simulink model "System_Stability_Evaluation"  (R2024a)
settings: Solver=VariableStepAuto  StartTime=0.0  StopTime=10.0  RelTol=1e-3
undefined symbols (not defined in the file or in its folder): sigbuilder_block
libraries: cstblocks x3
settings Model: Creator=marin  LastModifiedBy=marin

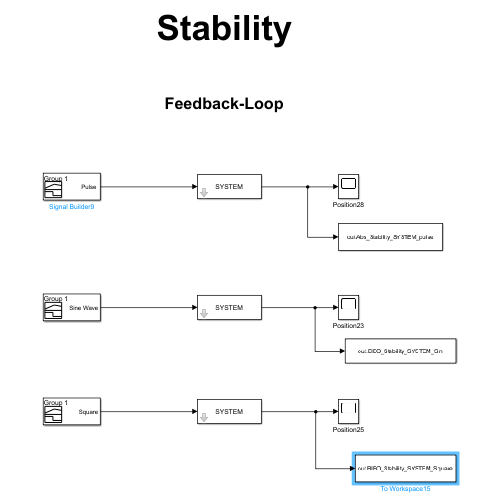
[thumbnail: Simulink's stored preview of the top-level diagram]
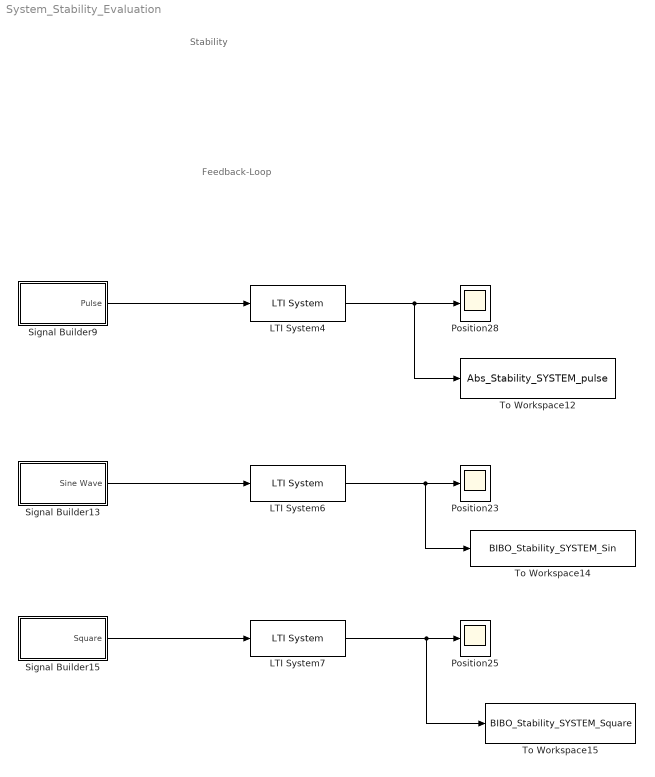
== system System_Stability_Evaluation ==
  note: Stability
  note: Feedback-Loop
  LTI System4 : cstblocks/LTI System  sys=SYSTEM  IC=[]  PadeOrder=0
  LTI System6 : cstblocks/LTI System  sys=SYSTEM  IC=[]  PadeOrder=0
  LTI System7 : cstblocks/LTI System  sys=SYSTEM  IC=[]  PadeOrder=0
  Position23 : Scope
  Position25 : Scope
  Position28 : Scope
  Signal Builder13 : Subsystem  Tag=STV Subsys  LoadFcn=sigbuilder_block('load');  StartFcn=sigbuilder_block('start');  StopFcn=sigbuilder_block('stop');  ClipboardFcn=sigbuilder_block('clipboard');  mask(Sigbuilder block){tuvar=[0:10]}
      mask help: Simulink:masks:SigbuilderBlock_MD
      mask init:
      | if ~strcmp(get_param(bdroot(gcbh),'SimulationStatus'),'stopped') tuvar = sigbuilder_block('maskInit'); end
      settings: CopyFcn=sigbuilder_block('copy');  DeleteFcn=sigbuilder_block('delete');  ModelCloseFcn=sigbuilder_block('modelClose');  PreSaveFcn=sigbuilder_block('preSave');  PauseFcn=sigbuilder_block('pause');  ContinueFcn=sigbuilder_block('continue');  NameChangeFcn=sigbuilder_block('namechange');  OpenFcn=sigbuilder_block('open',[404 117.5 550.5 362.5 ]);  CloseFcn=sigbuilder_block('close');
      mask Display: plot(0, 0, 100, 100,[2, 2, 32, 32, 2], [68, 8, 8, 68, 68],[32, 2], [38, 38], [32, 19, 2],[53, 60, 44], [32, 17, 17, 2],[16, 16, 31, 31]);txt = getActiveGroup(gcbh);text(2, 100, txt,'verticalAlignment', 'top');
  Signal Builder15 : Subsystem  Tag=STV Subsys  LoadFcn=sigbuilder_block('load');  StartFcn=sigbuilder_block('start');  StopFcn=sigbuilder_block('stop');  ClipboardFcn=sigbuilder_block('clipboard');  mask(Sigbuilder block){tuvar=[0:10]}
      mask help: Simulink:masks:SigbuilderBlock_MD
      mask init:
      | if ~strcmp(get_param(bdroot(gcbh),'SimulationStatus'),'stopped') tuvar = sigbuilder_block('maskInit'); end
      settings: CopyFcn=sigbuilder_block('copy');  DeleteFcn=sigbuilder_block('delete');  ModelCloseFcn=sigbuilder_block('modelClose');  PreSaveFcn=sigbuilder_block('preSave');  PauseFcn=sigbuilder_block('pause');  ContinueFcn=sigbuilder_block('continue');  NameChangeFcn=sigbuilder_block('namechange');  OpenFcn=sigbuilder_block('open',[404 117.5 550.5 362.5 ]);  CloseFcn=sigbuilder_block('close');
      mask Display: plot(0, 0, 100, 100,[2, 2, 32, 32, 2], [68, 8, 8, 68, 68],[32, 2], [38, 38], [32, 19, 2],[53, 60, 44], [32, 17, 17, 2],[16, 16, 31, 31]);txt = getActiveGroup(gcbh);text(2, 100, txt,'verticalAlignment', 'top');
  Signal Builder9 : Subsystem  Tag=STV Subsys  LoadFcn=sigbuilder_block('load');  StartFcn=sigbuilder_block('start');  StopFcn=sigbuilder_block('stop');  ClipboardFcn=sigbuilder_block('clipboard');  mask(Sigbuilder block){tuvar=[0:10]}
      mask help: Simulink:masks:SigbuilderBlock_MD
      mask init:
      | if ~strcmp(get_param(bdroot(gcbh),'SimulationStatus'),'stopped') tuvar = sigbuilder_block('maskInit'); end
      settings: CopyFcn=sigbuilder_block('copy');  DeleteFcn=sigbuilder_block('delete');  ModelCloseFcn=sigbuilder_block('modelClose');  PreSaveFcn=sigbuilder_block('preSave');  PauseFcn=sigbuilder_block('pause');  ContinueFcn=sigbuilder_block('continue');  NameChangeFcn=sigbuilder_block('namechange');  OpenFcn=sigbuilder_block('open',[404 117.5 550.5 362.5 ]);  CloseFcn=sigbuilder_block('close');
      mask Display: plot(0, 0, 100, 100,[2, 2, 32, 32, 2], [68, 8, 8, 68, 68],[32, 2], [38, 38], [32, 19, 2],[53, 60, 44], [32, 17, 17, 2],[16, 16, 31, 31]);txt = getActiveGroup(gcbh);text(2, 100, txt,'verticalAlignment', 'top');
  To Workspace12 : ToWorkspace  VariableName=Abs_Stability_SYSTEM_pulse  SampleTime=-1
  To Workspace14 : ToWorkspace  VariableName=BIBO_Stability_SYSTEM_Sin  SampleTime=-1
  To Workspace15 : ToWorkspace  VariableName=BIBO_Stability_SYSTEM_Square  SampleTime=-1
  wires:
  LTI System4/1 -> Position28/1, To Workspace12/1
  Signal Builder9/1("Pulse ") -> LTI System4/1
  Signal Builder15/1(Square) -> LTI System7/1
  LTI System7/1 -> Position25/1, To Workspace15/1
  LTI System6/1 -> Position23/1, To Workspace14/1
  Signal Builder13/1(Sine Wave) -> LTI System6/1

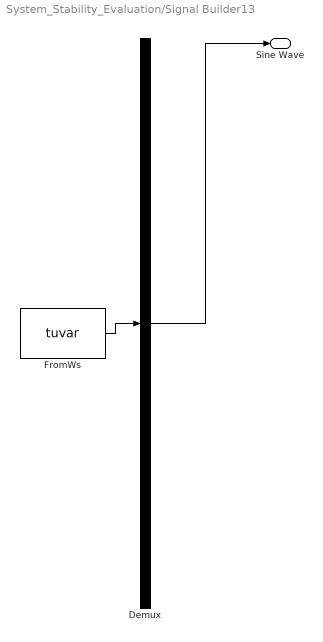
== system System_Stability_Evaluation/Signal Builder13 ==
  Demux : Demux  Tag=STV Demux  Outputs=1
      settings: DisplayOption=none
  FromWs : FromWorkspace  Tag=STV FromWs  VariableName=tuvar
      SigBuilderData=|
      | common.afterFinalStr = 'Extrapolate'
      | common.sampleTime = 0
      | dataSet.timeRange = [0 10]
      | dataSet.name = 'Group 1'
      | sbobj.Groups.Name = 'Group 1'
      | sbobj.Groups.Signals.Name = 'Sine Wave'
      | sbobj.Groups.Signals.XData = [0 0.111111111111 0.222222222222 0.333333333333 0.444444444444 0.555555555556 0.666666666667 0.777777777778 0.888888888889 1 1.11111111111 1.22222222222 1.33333333333 1.44444444444 1.55555555556 1.66666666667 1.77777777778 1.88888888889 2 2.11111111111 2.22222222222 2.33333333333 2.44444444444 2.55555555556 2.66666666667 2.77777777778 2.88888888889 3 3.11111111111 3.22222222222 3.33333333333 3.44444444444 3.55555555556 3.66666666667 3.77777777778 3.88888888889 4 4.11111111111 4.22222222222 4.33333333333 4.44444444444 4.55555555556 4.66666666667 4.77777777778 4.88888888889 5 5.11111111111 5.22222222222 5.33333333333 5.44444444444 5.55555555556 5.66666666667 5.77777777778 5.88888888889 6 6.11111111111 6.22222222222 6.33333333333 6.44444444444 6.55555555556 6.66666666667 6.77777777778 6.88888888889 7 7.11111111111 7.22222222222 7.33333333333 7.44444444444 7.55555555556 7.66666666667 7.77777777778 7.88888888889 8 8.11111111111 8.22222222222 8.33333333333 8.44444444444 8.55555555556 8.66666666667 8.77777777778 8.88888888889 9 9.11111111111 9.22222222222 9.33333333333 9.44444444444 9.55555555556 9.66666666667 9.77777777778 9.88888888889 10]
      | sbobj.Groups.Signals.YData = [1 1.64278760969 1.98480775301 1.86602540378 1.34202014333 0.657979856674 0.133974596216 0.0151922469878 0.357212390313 1 1.64278760969 1.98480775301 1.86602540378 1.34202014333 0.657979856674 0.133974596216 0.0151922469878 0.357212390313 1 1.64278760969 1.98480775301 1.86602540378 1.34202014333 0.657979856674 0.133974596216 0.0151922469878 0.357212390313 1 1.64278760969 1.98480775301 1.86602540378 1.34202014333 0.657979856674 0.133974596216 0.0151922469878 0.357212390313 1 1.64278760969 1.98480775301 1.86602540378 1.34202014333 0.657979856674 0.133974596216 0.0151922469878 0.357212390313 1 1.64278760969 1.98480775301 1.86602540378 1.34202014333 0.657979856674 0.133974596216 0.0151922469878 0.357212390313 1 1.64278760969 1.98480775301 1.86602540378 1.34202014333 0.657979856674 0.133974596216 0.0151922469878 0.357212390313 1 1.64278760969 1.98480775301 1.86602540378 1.34202014333 0.657979856674 0.133974596216 0.0151922469878 0.357212390313 1 1.64278760969 1.98480775301 1.86602540378 1.34202014333 0.657979856674 0.133974596216 0.0151922469878 0.357212390313 1 1.64278760969 1.98480775301 1.86602540378 1.34202014333 0.657979856674 0.133974596216 0.0151922469878 0.357212390313 1]
  Sine Wave : Outport  Tag=STV Outport
  wires:
  FromWs/1 -> Demux/1
  Demux/1 -> Sine Wave/1

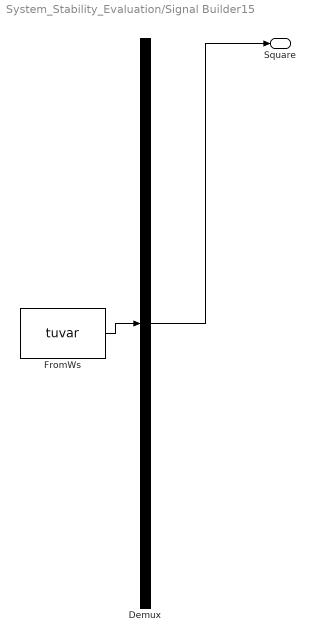
== system System_Stability_Evaluation/Signal Builder15 ==
  Demux : Demux  Tag=STV Demux  Outputs=1
      settings: DisplayOption=none
  FromWs : FromWorkspace  Tag=STV FromWs  VariableName=tuvar
      SigBuilderData=|
      | common.afterFinalStr = 'Extrapolate'
      | common.sampleTime = 0
      | dataSet.timeRange = [0 10]
      | dataSet.name = 'Group 1'
      | sbobj.Groups.Name = 'Group 1'
      | sbobj.Groups.Signals.Name = 'Square'
      | sbobj.Groups.Signals.XData = [0 0.5 0.5 1 1 1.5 1.5 2 2 2.5 2.5 3 3 3.5 3.5 4 4 4.5 4.5 5 5 5.5 5.5 6 6 6.5 6.5 7 7 7.5 7.5 8 8 8.5 8.5 9 9 9.5 9.5 10]
      | sbobj.Groups.Signals.YData = [2 2 0 0 2 2 0 0 2 2 0 0 2 2 0 0 2 2 0 0 2 2 0 0 2 2 0 0 2 2 0 0 2 2 0 0 2 2 0 0]
  Square : Outport  Tag=STV Outport
  wires:
  Demux/1 -> Square/1
  FromWs/1 -> Demux/1

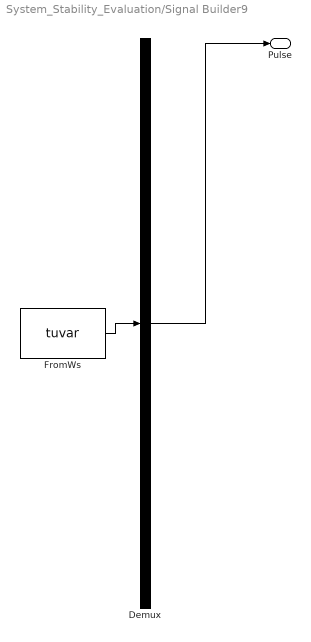
== system System_Stability_Evaluation/Signal Builder9 ==
  Demux : Demux  Tag=STV Demux  Outputs=1
      settings: DisplayOption=none
  FromWs : FromWorkspace  Tag=STV FromWs  VariableName=tuvar
      SigBuilderData=|
      | common.afterFinalStr = 'Extrapolate'
      | common.sampleTime = 0
      | dataSet.timeRange = [0 10]
      | dataSet.name = 'Group 1'
      | sbobj.Groups.Name = 'Group 1'
      | sbobj.Groups.Signals.Name = 'Pulse '
      | sbobj.Groups.Signals.XData = [0 4 4 6 6 10]
      | sbobj.Groups.Signals.YData = [0 0 1 1 0 0]
  "Pulse " : Outport  Tag=STV Outport
  wires:
  FromWs/1 -> Demux/1
  Demux/1 -> "Pulse "/1
